simulink model "MdSWReqChk358"  (R2018b)
settings: Solver=FixedStepDiscrete  StartTime=0.0  StopTime=10.0  FixedStep=0.01  RelTol=1e-3
undefined symbols (not defined in the file or in its folder): ChkBsyBitArray4s, ChkBsyBitArray6s7s, KeSMSAutoEZEFwdBkwdPosEna_Val, KeSMSuButtonLongPressedThrshldTm_Val, KeSMSuMdNum4s_Val, KeSMSuMdNum6s7s_Val, SetBsyBitArray4s, SetEnBitArray4s
libraries: RspLib x14, simulink x9
settings Model: Creator=sn2xws  LastModifiedBy=sn55gm
settings Model: ModifiedHistory=|
  | 2023.8.1 CR401790  增加模式21-26的请求
  | V2.1.0
  | 2023.9.18 bug 542961符号方向反了，<= 改为>=
  | V2.3.0
  | 2023.12.28  迎宾向后，条件改为或
  | 2025.2.24 V2.3.1 358MY26车型新增md33，md34，共存模式规则变更
settings DataIOCC: SaveFormat=StructureWithTime
settings OptimizationCC: DefaultParameterBehavior=Inlined  EnhancedBackFolding=on  PassReuseOutputArgsAs=Individual arguments  ZeroExternalMemoryAtStartup=off  ZeroInternalMemoryAtStartup=off  OptimizeBlockOrder=speed  DifferentSizesBufferReuse=on  OptimizationCustomize=off
settings DebuggingCC: ParameterTunabilityLossMsg=error
settings ModelReferenceCC: ModelReferenceNumInstancesAllowed=Single
settings SFSimCC: MATLABDynamicMemAlloc=off
settings RTWCC: SystemTargetFile=autosar.tlc  GenCodeOnly=on  TemplateMakefile=ert_default_tmf  Description=AUTOSAR  GenerateReport=on  IncludeHyperlinkInReport=on  LaunchReport=on  GenerateTraceInfo=on  GenerateTraceReport=on  GenerateTraceReportSl=on  GenerateTraceReportSf=on  GenerateTraceReportEml=on  GenerateCodeMetricsReport=on
settings CodeAppCC: ForceParamTrailComments=on  IgnoreCustomStorageClasses=off  OperatorAnnotations=on  SimulinkDataObjDesc=on  SFDataObjDesc=on  InsertBlockDesc=on
settings STFCustomTargetCC: TargetLangStandard=C99 (ISO)  MultiwordLength=256  ParMdlRefBuildCompliant=on  CompOptLevelCompliant=on  IncludeMdlTerminateFcn=off  CombineOutputUpdateFcns=on  SuppressErrorStatus=on  ERTCustomFileBanners=on  SupportNonFinite=off  SupportComplex=off  SupportContinuousTime=off  SupportNonInlinedSFcns=off  RemoveResetFunc=on  MATLABClassNameForMDSCustomization=Simulink.SoftwareTarget.ERTCustomization  AutosarCompliant=on  UseToolchainInfoCompliant=on  LookupTableObjectStructAxisOrder=2,1,3,4,...  LUTObjectStructOrderEvenSpacing=Size,Table,Breakpoints  SystemTargetFile=autosar.tlc
settings ERTTargetCC: TargetLangStandard=C99 (ISO)  ConcurrentExecutionCompliant=off  IncludeMdlTerminateFcn=off  SuppressErrorStatus=on  SupportNonFinite=off  SupportComplex=off  ModelStepFunctionPrototypeControlCompliant=off  CPPClassGenCompliant=off  AutosarCompliant=on  LookupTableObjectStructAxisOrder=2,1,3,4,...  LUTObjectStructOrderEvenSpacing=Size,Table,Breakpoints  InlinedParameterPlacement=NonHierarchical  ERTCustomFileTemplate=example_file_process.tlc  ERTFilePackagingFormat=Compact

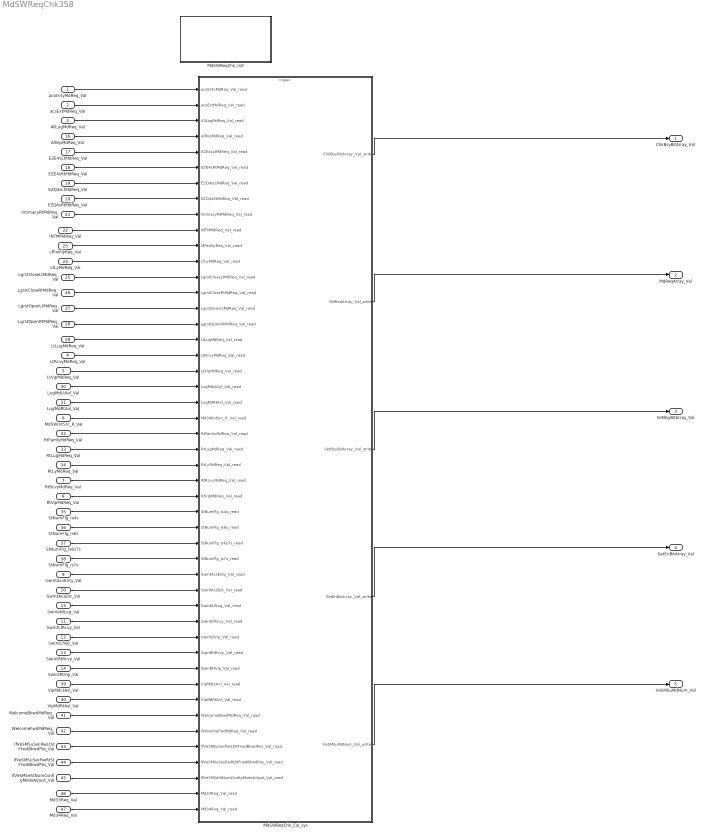
== system MdSWReqChk358 ==
  acsEntyMdReq_Val : Inport  OutDataTypeStr=boolean  PortDimensions=1
  acsExtMdReq_Val : Inport  Port=2  OutDataTypeStr=boolean  PortDimensions=1
  AllLugMdReq_Val : Inport  Port=3  OutDataTypeStr=boolean  PortDimensions=1
  LtRcvyMdReq_Val : Inport  Port=4  OutDataTypeStr=boolean  PortDimensions=1
  LtVipMdReq_Val : Inport  Port=5  OutDataTypeStr=boolean  PortDimensions=1
  MdSWIntSrc_R_Val : Inport  Port=6  OutDataTypeStr=uint16  PortDimensions=1
  RtRcvyMdReq_Val : Inport  Port=7  OutDataTypeStr=boolean  PortDimensions=1
  RtVipMdReq_Val : Inport  Port=8  OutDataTypeStr=boolean  PortDimensions=1
  SwIntAcsEnty_Val : Inport  Port=9  OutDataTypeStr=IntEnable  PortDimensions=1
  SwIntAcsExt_Val : Inport  Port=10  OutDataTypeStr=IntEnable  PortDimensions=1
  SwIntLfRcvy_Val : Inport  Port=11  OutDataTypeStr=IntEnable  PortDimensions=1
  SwIntLfVip_Val : Inport  Port=12  OutDataTypeStr=IntEnable  PortDimensions=1
  SwIntRtRcvy_Val : Inport  Port=13  OutDataTypeStr=IntEnable  PortDimensions=1
  SwIntRtVip_Val : Inport  Port=14  OutDataTypeStr=IntEnable  PortDimensions=1
  SwIntAllLug_Val : Inport  Port=15  OutDataTypeStr=IntEnable  PortDimensions=1
  AllVipMdReq_Val : Inport  Port=16  OutDataTypeStr=boolean  PortDimensions=1
  EZE4sLtMdReq_Val : Inport  Port=17  OutDataTypeStr=boolean  PortDimensions=1
  EZE4sRtMdReq_Val : Inport  Port=18  OutDataTypeStr=boolean  PortDimensions=1
  EZQ4sLtMdReq_Val : Inport  Port=19  OutDataTypeStr=boolean  PortDimensions=1
  EZQ4sRtMdReq_Val : Inport  Port=20  OutDataTypeStr=boolean  PortDimensions=1
  IntimacyRtMdReq_Val : Inport  Port=21  OutDataTypeStr=boolean  PortDimensions=1
  INTMMdReq_Val : Inport  Port=22  OutDataTypeStr=boolean  PortDimensions=1
  LfFamlyReq_Val : Inport  Port=23  OutDataTypeStr=boolean  PortDimensions=1
  LfLyMdReq_Val : Inport  Port=24  OutDataTypeStr=boolean  PortDimensions=1
  LgrstCloseLtMdReq_Val : Inport  Port=25  OutDataTypeStr=boolean  PortDimensions=1
  LgrstCloseRtMdReq_Val : Inport  Port=26  OutDataTypeStr=boolean  PortDimensions=1
  LgrstOpenLtMdReq_Val : Inport  Port=27  OutDataTypeStr=boolean  PortDimensions=1
  LgrstOpenRtMdReq_Val : Inport  Port=28  OutDataTypeStr=boolean  PortDimensions=1
  LtLugMdReq_Val : Inport  Port=29  OutDataTypeStr=boolean  PortDimensions=1
  LugMdLtAvl_Val : Inport  Port=30  OutDataTypeStr=boolean  PortDimensions=1
  LugMdRtAvl_Val : Inport  Port=31  OutDataTypeStr=boolean  PortDimensions=1
  RtFamlyMdReq_Val : Inport  Port=32  OutDataTypeStr=boolean  PortDimensions=1
  RtLugMdReq_Val : Inport  Port=33  OutDataTypeStr=boolean  PortDimensions=1
  RtLyMdReq_Val : Inport  Port=34  OutDataTypeStr=boolean  PortDimensions=1
  StNumFlg_Is4s : Inport  Port=35  OutDataTypeStr=boolean  PortDimensions=1
  StNumFlg_Is6s : Inport  Port=36  OutDataTypeStr=boolean  PortDimensions=1
  StNumFlg_Is6s7s : Inport  Port=37  OutDataTypeStr=boolean  PortDimensions=1
  StNumFlg_Is7s : Inport  Port=38  OutDataTypeStr=boolean  PortDimensions=1
  VipMdLtAvl_Val : Inport  Port=39  OutDataTypeStr=boolean  PortDimensions=1
  VipMdRtAvl_Val : Inport  Port=40  OutDataTypeStr=boolean  PortDimensions=1
  WelcomeBkwdMdReq_Val : Inport  Port=41  OutDataTypeStr=boolean  PortDimensions=1
  WelcomeFwdMdReq_Val : Inport  Port=42  OutDataTypeStr=boolean  PortDimensions=1
  IfVeSMSuSecRwLtStFrwdBkwdPos_Val : Inport  Port=43  OutDataTypeStr=uint16  PortDimensions=1
  IfVeSMSuSecRwRtStFrwdBkwdPos_Val : Inport  Port=44  OutDataTypeStr=uint16  PortDimensions=1
  IfVeSMSeStNumConfigModeAdjust_Val : Inport  Port=45  OutDataTypeStr=uint8  PortDimensions=1
  Md33Req_Val : Inport  Port=46  OutDataTypeStr=boolean  PortDimensions=1
  Md34Req_Val : Inport  Port=47  OutDataTypeStr=boolean  PortDimensions=1
  MdSWReqChk_Cal_sys : Subsystem
  MdSWReqChk_Init : Subsystem
  ChkBsyBitArray_Val : Outport  OutDataTypeStr=uint32  PortDimensions=32
  MdReqArray_Val : Outport  Port=2  OutDataTypeStr=boolean  PortDimensions=32
  SetBsyBitArray_Val : Outport  Port=3  OutDataTypeStr=uint32  PortDimensions=32
  SetEnBitArray_Val : Outport  Port=4  OutDataTypeStr=uint32  PortDimensions=32
  VeSMSuMdNum_Val : Outport  Port=5  OutDataTypeStr=uint8  PortDimensions=1
  wires:
  acsEntyMdReq_Val/1 -> MdSWReqChk_Cal_sys/1(acsEntyMdReq_Val_read)
  acsExtMdReq_Val/1 -> MdSWReqChk_Cal_sys/2(acsExtMdReq_Val_read)
  AllLugMdReq_Val/1 -> MdSWReqChk_Cal_sys/3(AllLugMdReq_Val_read)
  LtRcvyMdReq_Val/1 -> MdSWReqChk_Cal_sys/18(LtRcvyMdReq_Val_read)
  LtVipMdReq_Val/1 -> MdSWReqChk_Cal_sys/19(LtVipMdReq_Val_read)
  MdSWIntSrc_R_Val/1 -> MdSWReqChk_Cal_sys/22(MdSWIntSrc_R_Val_read)
  RtRcvyMdReq_Val/1 -> MdSWReqChk_Cal_sys/26(RtRcvyMdReq_Val_read)
  RtVipMdReq_Val/1 -> MdSWReqChk_Cal_sys/27(RtVipMdReq_Val_read)
  SwIntAcsEnty_Val/1 -> MdSWReqChk_Cal_sys/32(SwIntAcsEnty_Val_read)
  SwIntAcsExt_Val/1 -> MdSWReqChk_Cal_sys/33(SwIntAcsExt_Val_read)
  SwIntLfRcvy_Val/1 -> MdSWReqChk_Cal_sys/35(SwIntLfRcvy_Val_read)
  SwIntLfVip_Val/1 -> MdSWReqChk_Cal_sys/36(SwIntLfVip_Val_read)
  SwIntRtRcvy_Val/1 -> MdSWReqChk_Cal_sys/37(SwIntRtRcvy_Val_read)
  SwIntRtVip_Val/1 -> MdSWReqChk_Cal_sys/38(SwIntRtVip_Val_read)
  SwIntAllLug_Val/1 -> MdSWReqChk_Cal_sys/34(SwIntAllLug_Val_read)
  AllVipMdReq_Val/1 -> MdSWReqChk_Cal_sys/4(AllVipMdReq_Val_read)
  EZE4sLtMdReq_Val/1 -> MdSWReqChk_Cal_sys/5(EZE4sLtMdReq_Val_read)
  EZE4sRtMdReq_Val/1 -> MdSWReqChk_Cal_sys/6(EZE4sRtMdReq_Val_read)
  EZQ4sLtMdReq_Val/1 -> MdSWReqChk_Cal_sys/7(EZQ4sLtMdReq_Val_read)
  EZQ4sRtMdReq_Val/1 -> MdSWReqChk_Cal_sys/8(EZQ4sRtMdReq_Val_read)
  IntimacyRtMdReq_Val/1 -> MdSWReqChk_Cal_sys/9(IntimacyRtMdReq_Val_read)
  INTMMdReq_Val/1 -> MdSWReqChk_Cal_sys/10(INTMMdReq_Val_read)
  LfFamlyReq_Val/1 -> MdSWReqChk_Cal_sys/11(LfFamlyReq_Val_read)
  LfLyMdReq_Val/1 -> MdSWReqChk_Cal_sys/12(LfLyMdReq_Val_read)
  LgrstCloseLtMdReq_Val/1 -> MdSWReqChk_Cal_sys/13(LgrstCloseLtMdReq_Val_read)
  LgrstCloseRtMdReq_Val/1 -> MdSWReqChk_Cal_sys/14(LgrstCloseRtMdReq_Val_read)
  LgrstOpenLtMdReq_Val/1 -> MdSWReqChk_Cal_sys/15(LgrstOpenLtMdReq_Val_read)
  LgrstOpenRtMdReq_Val/1 -> MdSWReqChk_Cal_sys/16(LgrstOpenRtMdReq_Val_read)
  LtLugMdReq_Val/1 -> MdSWReqChk_Cal_sys/17(LtLugMdReq_Val_read)
  LugMdLtAvl_Val/1 -> MdSWReqChk_Cal_sys/20(LugMdLtAvl_Val_read)
  LugMdRtAvl_Val/1 -> MdSWReqChk_Cal_sys/21(LugMdRtAvl_Val_read)
  RtFamlyMdReq_Val/1 -> MdSWReqChk_Cal_sys/23(RtFamlyMdReq_Val_read)
  RtLugMdReq_Val/1 -> MdSWReqChk_Cal_sys/24(RtLugMdReq_Val_read)
  RtLyMdReq_Val/1 -> MdSWReqChk_Cal_sys/25(RtLyMdReq_Val_read)
  StNumFlg_Is4s/1 -> MdSWReqChk_Cal_sys/28(StNumFlg_Is4s_read)
  StNumFlg_Is6s/1 -> MdSWReqChk_Cal_sys/29(StNumFlg_Is6s_read)
  StNumFlg_Is6s7s/1 -> MdSWReqChk_Cal_sys/30(StNumFlg_Is6s7s_read)
  StNumFlg_Is7s/1 -> MdSWReqChk_Cal_sys/31(StNumFlg_Is7s_read)
  VipMdLtAvl_Val/1 -> MdSWReqChk_Cal_sys/39(VipMdLtAvl_Val_read)
  VipMdRtAvl_Val/1 -> MdSWReqChk_Cal_sys/40(VipMdRtAvl_Val_read)
  WelcomeBkwdMdReq_Val/1 -> MdSWReqChk_Cal_sys/41(WelcomeBkwdMdReq_Val_read)
  WelcomeFwdMdReq_Val/1 -> MdSWReqChk_Cal_sys/42(WelcomeFwdMdReq_Val_read)
  MdSWReqChk_Cal_sys/1(ChkBsyBitArray_Val_write) -> ChkBsyBitArray_Val/1
  MdSWReqChk_Cal_sys/2(MdReqArray_Val_write) -> MdReqArray_Val/1
  MdSWReqChk_Cal_sys/3(SetBsyBitArray_Val_write) -> SetBsyBitArray_Val/1
  MdSWReqChk_Cal_sys/4(SetEnBitArray_Val_write) -> SetEnBitArray_Val/1
  MdSWReqChk_Cal_sys/5(VeSMSuMdNum_Val_write) -> VeSMSuMdNum_Val/1
  IfVeSMSuSecRwLtStFrwdBkwdPos_Val/1 -> MdSWReqChk_Cal_sys/43(IfVeSMSuSecRwLtStFrwdBkwdPos_Val_read)
  IfVeSMSuSecRwRtStFrwdBkwdPos_Val/1 -> MdSWReqChk_Cal_sys/44(IfVeSMSuSecRwRtStFrwdBkwdPos_Val_read)
  IfVeSMSeStNumConfigModeAdjust_Val/1 -> MdSWReqChk_Cal_sys/45(IfVeSMSeStNumConfigModeAdjust_Val_read)
  Md33Req_Val/1 -> MdSWReqChk_Cal_sys/46(Md33Req_Val_read)
  Md34Req_Val/1 -> MdSWReqChk_Cal_sys/47(Md34Req_Val_read)

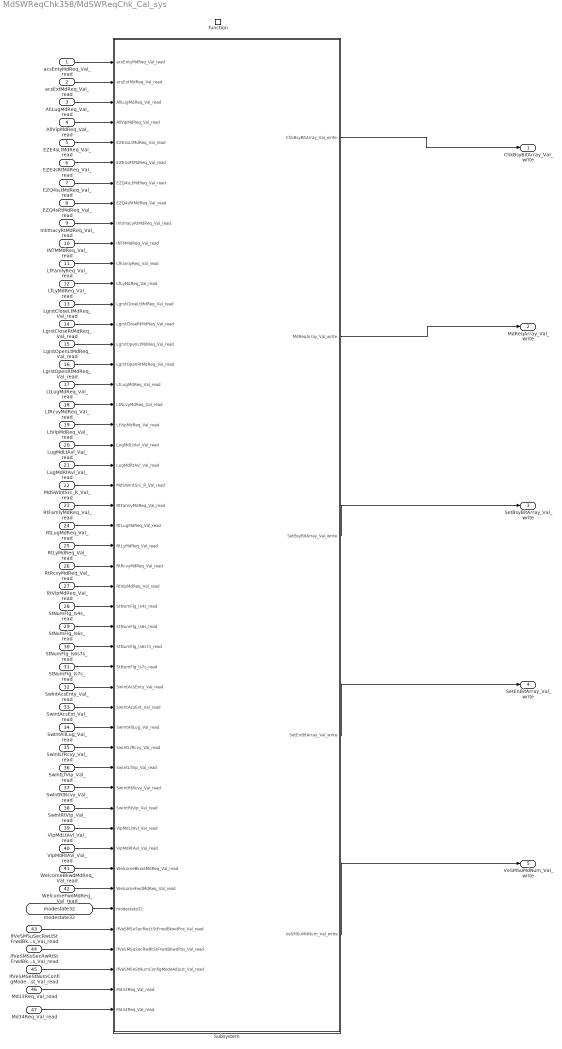
== system MdSWReqChk358/MdSWReqChk_Cal_sys ==
  acsEntyMdReq_Val_read : Inport
  acsExtMdReq_Val_read : Inport  Port=2
  AllLugMdReq_Val_read : Inport  Port=3
  AllVipMdReq_Val_read : Inport  Port=4
  EZE4sLtMdReq_Val_read : Inport  Port=5
  EZE4sRtMdReq_Val_read : Inport  Port=6
  EZQ4sLtMdReq_Val_read : Inport  Port=7
  EZQ4sRtMdReq_Val_read : Inport  Port=8
  IntimacyRtMdReq_Val_read : Inport  Port=9
  INTMMdReq_Val_read : Inport  Port=10
  LfFamlyReq_Val_read : Inport  Port=11
  LfLyMdReq_Val_read : Inport  Port=12
  LgrstCloseLtMdReq_Val_read : Inport  Port=13
  LgrstCloseRtMdReq_Val_read : Inport  Port=14
  LgrstOpenLtMdReq_Val_read : Inport  Port=15
  LgrstOpenRtMdReq_Val_read : Inport  Port=16
  LtLugMdReq_Val_read : Inport  Port=17
  LtRcvyMdReq_Val_read : Inport  Port=18
  LtVipMdReq_Val_read : Inport  Port=19
  LugMdLtAvl_Val_read : Inport  Port=20
  LugMdRtAvl_Val_read : Inport  Port=21
  MdSWIntSrc_R_Val_read : Inport  Port=22
  RtFamlyMdReq_Val_read : Inport  Port=23
  RtLugMdReq_Val_read : Inport  Port=24
  RtLyMdReq_Val_read : Inport  Port=25
  RtRcvyMdReq_Val_read : Inport  Port=26
  RtVipMdReq_Val_read : Inport  Port=27
  StNumFlg_Is4s_read : Inport  Port=28
  StNumFlg_Is6s_read : Inport  Port=29
  StNumFlg_Is6s7s_read : Inport  Port=30
  StNumFlg_Is7s_read : Inport  Port=31
  SwIntAcsEnty_Val_read : Inport  Port=32
  SwIntAcsExt_Val_read : Inport  Port=33
  SwIntAllLug_Val_read : Inport  Port=34
  SwIntLfRcvy_Val_read : Inport  Port=35
  SwIntLfVip_Val_read : Inport  Port=36
  SwIntRtRcvy_Val_read : Inport  Port=37
  SwIntRtVip_Val_read : Inport  Port=38
  VipMdLtAvl_Val_read : Inport  Port=39
  VipMdRtAvl_Val_read : Inport  Port=40
  WelcomeBkwdMdReq_Val_read : Inport  Port=41
  WelcomeFwdMdReq_Val_read : Inport  Port=42
  IfVeSMSuSecRwLtStFrwdBkwdPos_Val_read : Inport  Port=43
  IfVeSMSuSecRwRtStFrwdBkwdPos_Val_read : Inport  Port=44
  IfVeSMSeStNumConfigModeAdjust_Val_read : Inport  Port=45
  Md33Req_Val_read : Inport  Port=46
  Md34Req_Val_read : Inport  Port=47
  function : TriggerPort  TriggerType=function-call  IsSimulinkFunction=on  FunctionName=MdSWReqChk_Cal  VariantControl=(inherit)
  Subsystem : Subsystem
  modestate32 : ArgIn  OutDataTypeStr=uint32  ArgumentName=modestate32
  ChkBsyBitArray_Val_write : Outport
      settings: EnsureOutportIsVirtual=on
  MdReqArray_Val_write : Outport  Port=2
      settings: EnsureOutportIsVirtual=on
  SetBsyBitArray_Val_write : Outport  Port=3
      settings: EnsureOutportIsVirtual=on
  SetEnBitArray_Val_write : Outport  Port=4
      settings: EnsureOutportIsVirtual=on
  VeSMSuMdNum_Val_write : Outport  Port=5
      settings: EnsureOutportIsVirtual=on
  wires:
  acsEntyMdReq_Val_read/1 -> Subsystem/1(acsEntyMdReq_Val_read)
  acsExtMdReq_Val_read/1 -> Subsystem/2(acsExtMdReq_Val_read)
  AllLugMdReq_Val_read/1 -> Subsystem/3(AllLugMdReq_Val_read)
  AllVipMdReq_Val_read/1 -> Subsystem/4(AllVipMdReq_Val_read)
  EZE4sLtMdReq_Val_read/1 -> Subsystem/5(EZE4sLtMdReq_Val_read)
  EZE4sRtMdReq_Val_read/1 -> Subsystem/6(EZE4sRtMdReq_Val_read)
  EZQ4sLtMdReq_Val_read/1 -> Subsystem/7(EZQ4sLtMdReq_Val_read)
  EZQ4sRtMdReq_Val_read/1 -> Subsystem/8(EZQ4sRtMdReq_Val_read)
  IntimacyRtMdReq_Val_read/1 -> Subsystem/9(IntimacyRtMdReq_Val_read)
  INTMMdReq_Val_read/1 -> Subsystem/10(INTMMdReq_Val_read)
  LfFamlyReq_Val_read/1 -> Subsystem/11(LfFamlyReq_Val_read)
  LfLyMdReq_Val_read/1 -> Subsystem/12(LfLyMdReq_Val_read)
  LgrstCloseLtMdReq_Val_read/1 -> Subsystem/13(LgrstCloseLtMdReq_Val_read)
  LgrstCloseRtMdReq_Val_read/1 -> Subsystem/14(LgrstCloseRtMdReq_Val_read)
  LgrstOpenLtMdReq_Val_read/1 -> Subsystem/15(LgrstOpenLtMdReq_Val_read)
  LgrstOpenRtMdReq_Val_read/1 -> Subsystem/16(LgrstOpenRtMdReq_Val_read)
  LtLugMdReq_Val_read/1 -> Subsystem/17(LtLugMdReq_Val_read)
  LtRcvyMdReq_Val_read/1 -> Subsystem/18(LtRcvyMdReq_Val_read)
  LtVipMdReq_Val_read/1 -> Subsystem/19(LtVipMdReq_Val_read)
  LugMdLtAvl_Val_read/1 -> Subsystem/20(LugMdLtAvl_Val_read)
  LugMdRtAvl_Val_read/1 -> Subsystem/21(LugMdRtAvl_Val_read)
  MdSWIntSrc_R_Val_read/1 -> Subsystem/22(MdSWIntSrc_R_Val_read)
  RtFamlyMdReq_Val_read/1 -> Subsystem/23(RtFamlyMdReq_Val_read)
  RtLugMdReq_Val_read/1 -> Subsystem/24(RtLugMdReq_Val_read)
  RtLyMdReq_Val_read/1 -> Subsystem/25(RtLyMdReq_Val_read)
  RtRcvyMdReq_Val_read/1 -> Subsystem/26(RtRcvyMdReq_Val_read)
  RtVipMdReq_Val_read/1 -> Subsystem/27(RtVipMdReq_Val_read)
  StNumFlg_Is4s_read/1 -> Subsystem/28(StNumFlg_Is4s_read)
  StNumFlg_Is6s_read/1 -> Subsystem/29(StNumFlg_Is6s_read)
  StNumFlg_Is6s7s_read/1 -> Subsystem/30(StNumFlg_Is6s7s_read)
  StNumFlg_Is7s_read/1 -> Subsystem/31(StNumFlg_Is7s_read)
  SwIntAcsEnty_Val_read/1 -> Subsystem/32(SwIntAcsEnty_Val_read)
  SwIntAcsExt_Val_read/1 -> Subsystem/33(SwIntAcsExt_Val_read)
  SwIntAllLug_Val_read/1 -> Subsystem/34(SwIntAllLug_Val_read)
  SwIntLfRcvy_Val_read/1 -> Subsystem/35(SwIntLfRcvy_Val_read)
  SwIntLfVip_Val_read/1 -> Subsystem/36(SwIntLfVip_Val_read)
  SwIntRtRcvy_Val_read/1 -> Subsystem/37(SwIntRtRcvy_Val_read)
  SwIntRtVip_Val_read/1 -> Subsystem/38(SwIntRtVip_Val_read)
  VipMdLtAvl_Val_read/1 -> Subsystem/39(VipMdLtAvl_Val_read)
  VipMdRtAvl_Val_read/1 -> Subsystem/40(VipMdRtAvl_Val_read)
  WelcomeBkwdMdReq_Val_read/1 -> Subsystem/41(WelcomeBkwdMdReq_Val_read)
  WelcomeFwdMdReq_Val_read/1 -> Subsystem/42(WelcomeFwdMdReq_Val_read)
  Subsystem/1(ChkBsyBitArray_Val_write) -> ChkBsyBitArray_Val_write/1
  Subsystem/2(MdReqArray_Val_write) -> MdReqArray_Val_write/1
  Subsystem/3(SetBsyBitArray_Val_write) -> SetBsyBitArray_Val_write/1
  Subsystem/4(SetEnBitArray_Val_write) -> SetEnBitArray_Val_write/1
  modestate32/1 -> Subsystem/43(modestate32)
  Subsystem/5(VeSMSuMdNum_Val_write) -> VeSMSuMdNum_Val_write/1
  IfVeSMSuSecRwLtStFrwdBkwdPos_Val_read/1 -> Subsystem/44(IfVeSMSuSecRwLtStFrwdBkwdPos_Val_read)
  IfVeSMSuSecRwRtStFrwdBkwdPos_Val_read/1 -> Subsystem/45(IfVeSMSuSecRwRtStFrwdBkwdPos_Val_read)
  IfVeSMSeStNumConfigModeAdjust_Val_read/1 -> Subsystem/46(IfVeSMSeStNumConfigModeAdjust_Val_read)
  Md33Req_Val_read/1 -> Subsystem/47(Md33Req_Val_read)
  Md34Req_Val_read/1 -> Subsystem/48(Md34Req_Val_read)

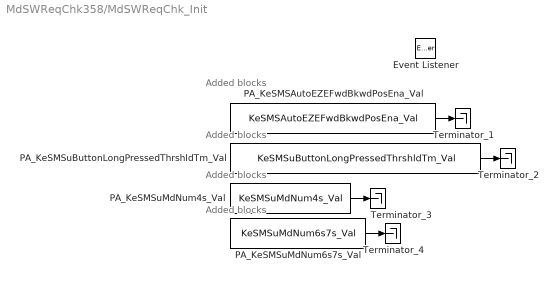
== system MdSWReqChk358/MdSWReqChk_Init ==
  note: Added blocks
  note: Added blocks
  note: Added blocks
  note: Added blocks
  Event Listener : EventListener  EventName=reset
  PA_KeSMSAutoEZEFwdBkwdPosEna_Val : Constant  Value=KeSMSAutoEZEFwdBkwdPosEna_Val
  PA_KeSMSuButtonLongPressedThrshldTm_Val : Constant  Value=KeSMSuButtonLongPressedThrshldTm_Val
  PA_KeSMSuMdNum4s_Val : Constant  Value=KeSMSuMdNum4s_Val
  PA_KeSMSuMdNum6s7s_Val : Constant  Value=KeSMSuMdNum6s7s_Val
  Terminator_{1..4} (4 alike) : Terminator
  wires:
  PA_KeSMSAutoEZEFwdBkwdPosEna_Val/1 -> Terminator_1/1
  PA_KeSMSuButtonLongPressedThrshldTm_Val/1 -> Terminator_2/1
  PA_KeSMSuMdNum4s_Val/1 -> Terminator_3/1
  PA_KeSMSuMdNum6s7s_Val/1 -> Terminator_4/1

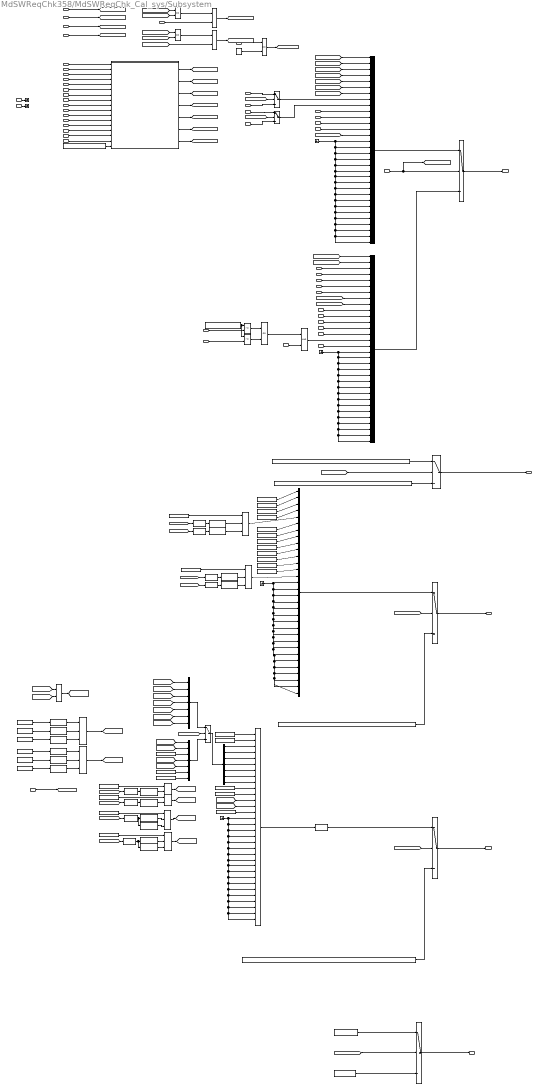
== system MdSWReqChk358/MdSWReqChk_Cal_sys/Subsystem ==
  note: 2023.12.28 迎宾向后，条件改为或
  note: bug542961
  note: 符号方向反了，<= 改为>=
  note: 2023.8.1 CR401790 增加模式21-26的请求
  note: VIPR
  note: RcvyR
  note: VIPL
  note: LugL
  note: LugR
  note: RcvyL
  acsEntyMdReq_Val_read : Inport
  acsExtMdReq_Val_read : Inport  Port=2
  AllLugMdReq_Val_read : Inport  Port=3
  AllVipMdReq_Val_read : Inport  Port=4
  EZE4sLtMdReq_Val_read : Inport  Port=5
  EZE4sRtMdReq_Val_read : Inport  Port=6
  EZQ4sLtMdReq_Val_read : Inport  Port=7
  EZQ4sRtMdReq_Val_read : Inport  Port=8
  IntimacyRtMdReq_Val_read : Inport  Port=9
  INTMMdReq_Val_read : Inport  Port=10
  LfFamlyReq_Val_read : Inport  Port=11
  LfLyMdReq_Val_read : Inport  Port=12
  LgrstCloseLtMdReq_Val_read : Inport  Port=13
  LgrstCloseRtMdReq_Val_read : Inport  Port=14
  LgrstOpenLtMdReq_Val_read : Inport  Port=15
  LgrstOpenRtMdReq_Val_read : Inport  Port=16
  LtLugMdReq_Val_read : Inport  Port=17
  LtRcvyMdReq_Val_read : Inport  Port=18
  LtVipMdReq_Val_read : Inport  Port=19
  LugMdLtAvl_Val_read : Inport  Port=20
  LugMdRtAvl_Val_read : Inport  Port=21
  MdSWIntSrc_R_Val_read : Inport  Port=22
  RtFamlyMdReq_Val_read : Inport  Port=23
  RtLugMdReq_Val_read : Inport  Port=24
  RtLyMdReq_Val_read : Inport  Port=25
  RtRcvyMdReq_Val_read : Inport  Port=26
  RtVipMdReq_Val_read : Inport  Port=27
  StNumFlg_Is4s_read : Inport  Port=28
  StNumFlg_Is6s_read : Inport  Port=29
  StNumFlg_Is6s7s_read : Inport  Port=30
  StNumFlg_Is7s_read : Inport  Port=31
  SwIntAcsEnty_Val_read : Inport  Port=32
  SwIntAcsExt_Val_read : Inport  Port=33
  SwIntAllLug_Val_read : Inport  Port=34
  SwIntLfRcvy_Val_read : Inport  Port=35
  SwIntLfVip_Val_read : Inport  Port=36
  SwIntRtRcvy_Val_read : Inport  Port=37
  SwIntRtVip_Val_read : Inport  Port=38
  VipMdLtAvl_Val_read : Inport  Port=39
  VipMdRtAvl_Val_read : Inport  Port=40
  WelcomeBkwdMdReq_Val_read : Inport  Port=41
  WelcomeFwdMdReq_Val_read : Inport  Port=42
  modestate32 : Inport  Port=43
  IfVeSMSuSecRwLtStFrwdBkwdPos_Val_read : Inport  Port=44
  IfVeSMSuSecRwRtStFrwdBkwdPos_Val_read : Inport  Port=45
  IfVeSMSeStNumConfigModeAdjust_Val_read : Inport  Port=46
  Md33Req_Val_read : Inport  Port=47
  Md34Req_Val_read : Inport  Port=48
  Bitwise Operator{,1,4..7} (6 alike) : simulink/Logic and Bit Operations/Bitwise Operator  logicop=OR  UseBitMask=off  NumInputPorts=3  BitMask=bin2dec('11011001')  BitMaskRealWorld=Stored Integer
  Bitwise Operator2 : simulink/Logic and Bit Operations/Bitwise Operator  logicop=OR  UseBitMask=off  NumInputPorts=2  BitMask=bin2dec('11011001')  BitMaskRealWorld=Stored Integer
  Bitwise Operator3 : simulink/Logic and Bit Operations/Bitwise Operator  logicop=OR  UseBitMask=off  NumInputPorts=2  BitMask=bin2dec('11011001')  BitMaskRealWorld=Stored Integer
  Bitwise Operator8 : simulink/Logic and Bit Operations/Bitwise Operator  logicop=OR  UseBitMask=off  NumInputPorts=2  BitMask=bin2dec('11011001')  BitMaskRealWorld=Stored Integer
  Constant : Constant  Value=ChkBsyBitArray6s7s  OutDataTypeStr=uint32
  Constant1 : Constant  Value=ChkBsyBitArray4s  OutDataTypeStr=uint32
  Constant{4..6,8..10,39} (7 alike) : Constant  OutDataTypeStr=uint32
  Constant2 : Constant  Value=SetEnBitArray4s  OutDataTypeStr=uint32
  Constant26 : Constant  Value=8  OutDataTypeStr=uint32
  Constant27 : Constant  Value=512  OutDataTypeStr=uint32
  Constant28 : Constant  Value=2048  OutDataTypeStr=uint32
  Constant29 : Constant  Value=2  OutDataTypeStr=uint32
  Constant3 : Constant  Value=4
  Constant30 : Constant  Value=1024  OutDataTypeStr=uint32
  Constant31 : Constant  Value=4096  OutDataTypeStr=uint32
  Constant32 : Constant  Value=64  OutDataTypeStr=uint32
  Constant33 : Constant  Value=32  OutDataTypeStr=uint32
  Constant34 : Constant  Value=16  OutDataTypeStr=uint32
  Constant35 : Constant  Value=524288  OutDataTypeStr=uint32
  Constant36 : Constant  Value=128  OutDataTypeStr=uint32
  Constant37 : Constant  Value=256  OutDataTypeStr=uint32
  Constant38 : Constant  Value=4  OutDataTypeStr=uint32
  Constant{40..41,44..49} (8 alike) : Constant  Value=532479  OutDataTypeStr=uint32
  Constant42 : Constant  Value=526079  OutDataTypeStr=uint32
  Constant43 : Constant  Value=530815  OutDataTypeStr=uint32
  Constant50 : Constant  Value=526079  OutDataTypeStr=uint32
  Constant51 : Constant  Value=530815  OutDataTypeStr=uint32
  Constant7 : Constant  Value=SetBsyBitArray4s  OutDataTypeStr=uint32
  Data Type Conversion{,1..7} (8 alike) : DataTypeConversion  OutDataTypeStr=uint32
  Data Type Conversion11 : DataTypeConversion
  Demux : Demux  Outputs=7
  Ground{,1..3} (4 alike) : Ground
  Logical Operator : Logic  Operator=OR  AllPortsSameDT=off  OutDataTypeStr=boolean
  Logical Operator1 : Logic  AllPortsSameDT=off  OutDataTypeStr=boolean
  Logical Operator2 : Logic  Operator=OR  AllPortsSameDT=off  OutDataTypeStr=boolean
  Logical Operator3 : Logic  AllPortsSameDT=off  OutDataTypeStr=boolean
  Logical Operator4 : Logic  Operator=OR  AllPortsSameDT=off  OutDataTypeStr=boolean
  Logical Operator5 : Logic  AllPortsSameDT=off  OutDataTypeStr=boolean
  Mux{,1..3} (4 alike) : Mux  Inputs=32
  Mux4 : Mux  Inputs=7
  Mux5 : Mux  Inputs=7
  PA_KeSMSAutoEZEFwdBkwdPosEna_Val : Constant  Value=KeSMSAutoEZEFwdBkwdPosEna_Val
  PA_KeSMSuButtonLongPressedThrshldTm_Val : Constant  Value=KeSMSuButtonLongPressedThrshldTm_Val
  PA_KeSMSuMdNum4s_Val : Constant  Value=KeSMSuMdNum4s_Val
  PA_KeSMSuMdNum6s7s_Val : Constant  Value=KeSMSuMdNum6s7s_Val
  Relational Operator : RelationalOperator  OutDataTypeStr=boolean  RndMeth=Simplest
  Relational Operator1 : RelationalOperator  OutDataTypeStr=boolean  RndMeth=Simplest
  Relational Operator2 : RelationalOperator  Operator===  OutDataTypeStr=boolean  RndMeth=Simplest
  Shift Arithmetic : ArithShift  BitShiftNumber=9  BitShiftDirection=Left
  Shift Arithmetic1 : ArithShift  BitShiftNumber=11  BitShiftDirection=Left
  Shift Arithmetic10 : ArithShift  BitShiftNumber=10  BitShiftDirection=Left
  Shift Arithmetic11 : ArithShift  BitShiftNumber=9  BitShiftDirection=Left
  Shift Arithmetic12 : ArithShift  BitShiftNumber=5  BitShiftDirection=Left
  Shift Arithmetic13 : ArithShift  BitShiftNumber=6  BitShiftDirection=Left
  Shift Arithmetic14 : ArithShift  BitShiftNumber=11  BitShiftDirection=Left
  Shift Arithmetic15 : ArithShift  BitShiftNumber=12  BitShiftDirection=Left
  Shift Arithmetic2 : ArithShift  BitShiftNumber=7  BitShiftDirection=Left
  Shift Arithmetic3 : ArithShift  BitShiftNumber=8  BitShiftDirection=Left
  Shift Arithmetic4 : ArithShift  BitShiftNumber=8  BitShiftDirection=Left
  Shift Arithmetic5 : ArithShift  BitShiftNumber=7  BitShiftDirection=Left
  Shift Arithmetic6 : ArithShift  BitShiftNumber=12  BitShiftDirection=Left
  Shift Arithmetic7 : ArithShift  BitShiftNumber=10  BitShiftDirection=Left
  Shift Arithmetic8 : ArithShift  BitShiftNumber=11  BitShiftDirection=Left
  Shift Arithmetic9 : ArithShift  BitShiftNumber=9  BitShiftDirection=Left
  Subsystem : Subsystem
  Switch{,1..7} (8 alike) : Switch  Criteria=u2 > Threshold
  Terminator_28 : Terminator
  Terminator_29 : Terminator
  ChkBsyBitArray_Val_write : Outport
      settings: EnsureOutportIsVirtual=on
  MdReqArray_Val_write : Outport  Port=2
      settings: EnsureOutportIsVirtual=on
  SetBsyBitArray_Val_write : Outport  Port=3
      settings: EnsureOutportIsVirtual=on
  SetEnBitArray_Val_write : Outport  Port=4
      settings: EnsureOutportIsVirtual=on
  VeSMSuMdNum_Val_write : Outport  Port=5
      settings: EnsureOutportIsVirtual=on
  wires:
  StNumFlg_Is4s_read/1 -> Terminator_28/1
  StNumFlg_Is7s_read/1 -> [is7s]
  PA_KeSMSuButtonLongPressedThrshldTm_Val/1 -> Subsystem/17(KeSMSuButtonLongPressedThrshldTm_Val)
  StNumFlg_Is6s_read/1 -> Terminator_29/1
  modestate32/1 -> Subsystem/7(modestate32_Val_read)
  acsEntyMdReq_Val_read/1 -> Subsystem/1(acsEntyMdReq_Val_read)
  AllLugMdReq_Val_read/1 -> Subsystem/3(AllLugMdReq_Val_read)
  acsExtMdReq_Val_read/1 -> Subsystem/2(acsExtMdReq_Val_read)
  MdSWIntSrc_R_Val_read/1 -> Subsystem/6(MdSWIntSrc_R_Val_read)
  LtVipMdReq_Val_read/1 -> Subsystem/5(LtVipMdReq_Val_read)
  LtRcvyMdReq_Val_read/1 -> Subsystem/4(LtRcvyMdReq_Val_read)
  RtRcvyMdReq_Val_read/1 -> Subsystem/8(RtRcvyMdReq_Val_read)
  RtVipMdReq_Val_read/1 -> Subsystem/9(RtVipMdReq_Val_read)
  SwIntAcsEnty_Val_read/1 -> Subsystem/10(SwIntAcsEnty_Val_read)
  SwIntAcsExt_Val_read/1 -> Subsystem/11(SwIntAcsExt_Val_read)
  SwIntLfRcvy_Val_read/1 -> Subsystem/12(SwIntLfRcvy_Val_read)
  SwIntLfVip_Val_read/1 -> Subsystem/13(SwIntLfVip_Val_read)
  SwIntRtVip_Val_read/1 -> Subsystem/15(SwIntRtVip_Val_read)
  SwIntAllLug_Val_read/1 -> Subsystem/16(SwIntAllLug_Val_read)
  SwIntRtRcvy_Val_read/1 -> Subsystem/14(SwIntRtRcvy_Val_read)
  Subsystem/1(acsEntyMdReqChk_Val_write) -> [EZEReq]
  Subsystem/2(acsExtMdReqChk_Val_write) -> [EZQReq]
  Subsystem/3(AllLugMdReqChk_Val_write) -> [AllLugReq]
  Subsystem/4(LtRcvyMdReqChk_Val_write) -> [LtRcvyReq]
  Subsystem/5(LtVipMdReqChk_Val_write) -> [LtVIPReq]
  Subsystem/6(RtRcvyMdReqChk_Val_write) -> [RtRcvyReq]
  Subsystem/7(RtVipMdReqChk_Val_write) -> [RtVIPReq]
  [EZEReq] -> Mux/1
  [EZQReq] -> Mux/2
  [LtVIPReq] -> Mux/3
  [RtVIPReq] -> Mux/4
  VipMdLtAvl_Val_read/1 -> [VipLtAvl]
  VipMdRtAvl_Val_read/1 -> [VipRtAvl]
  [VipLtAvl] -> Logical Operator/1
  [VipRtAvl] -> Logical Operator/2
  Logical Operator/1 -> Logical Operator1/1
  AllVipMdReq_Val_read/1 -> Logical Operator1/2
  Logical Operator1/1 -> [AllVipReq]
  [AllVipReq] -> Mux/5
  [LtRcvyReq] -> Mux/6
  [RtRcvyReq] -> Mux/7
  INTMMdReq_Val_read/1 -> Mux/10
  IntimacyRtMdReq_Val_read/1 -> Mux/11
  LtLugMdReq_Val_read/1 -> Mux/12
  RtLugMdReq_Val_read/1 -> Mux/13
  Logical Operator3/1 -> [AllLugReqComfirm]
  [AllLugReq] -> Logical Operator3/2
  Logical Operator2/1 -> Logical Operator3/1
  LugMdLtAvl_Val_read/1 -> [LugLtAvl]
  LugMdRtAvl_Val_read/1 -> [LugRtAvl]
  [LugLtAvl] -> Logical Operator2/1
  [LugRtAvl] -> Logical Operator2/2
  [AllLugReqComfirm] -> Mux/14
  Switch/1 -> MdReqArray_Val_write/1
  StNumFlg_Is6s7s_read/1 -> [Is6s7s], Switch/2
  Mux/1 -> Switch/1
  Ground/1 -> Mux/32, Mux/31, Mux/30, Mux/29, Mux/28, Mux/27, Mux/26, Mux/25, Mux/24, Mux/23, Mux/22, Mux/21, Mux/20, Mux/19, Mux/18, Mux/17, Mux/16, Mux/15
  [LtVIPReq] -> Mux1/1
  [LtRcvyReq] -> Mux1/2
  LfLyMdReq_Val_read/1 -> Mux1/3
  LgrstOpenLtMdReq_Val_read/1 -> Mux1/4
  LgrstCloseLtMdReq_Val_read/1 -> Mux1/5
  EZE4sLtMdReq_Val_read/1 -> Mux1/6
  EZQ4sLtMdReq_Val_read/1 -> Mux1/7
  [RtVIPReq] -> Mux1/8
  [RtRcvyReq] -> Mux1/9
  RtLyMdReq_Val_read/1 -> Mux1/10
  LgrstOpenRtMdReq_Val_read/1 -> Mux1/11
  LgrstCloseRtMdReq_Val_read/1 -> Mux1/12
  EZE4sRtMdReq_Val_read/1 -> Mux1/13
  EZQ4sRtMdReq_Val_read/1 -> Mux1/14
  WelcomeFwdMdReq_Val_read/1 -> Mux1/16
  Ground1/1 -> Mux1/27, Mux1/28, Mux1/32, Mux1/31, Mux1/30, Mux1/29, Mux1/26, Mux1/25, Mux1/24, Mux1/23, Mux1/22, Mux1/21, Mux1/20, Mux1/19, Mux1/18, Mux1/17
  Mux1/1 -> Switch/3
  [Is6s7s] -> Switch1/2
  Switch1/1 -> ChkBsyBitArray_Val_write/1
  Constant/1 -> Switch1/1
  Constant1/1 -> Switch1/3
  Constant2/1 -> Switch2/3
  [Is6s7s] -> Switch2/2
  Constant33/1 -> Mux2/9
  Mux2/1 -> Switch2/1  "SetEnBitArray"
  Data Type Conversion/1 -> Shift Arithmetic/1
  Constant37/1 -> Mux2/13
  Constant39/1 -> Mux2/1
  [VipRtAvl] -> Data Type Conversion1/1
  Constant28/1 -> Mux2/4
  Constant26/1 -> Mux2/2
  Bitwise Operator/1 -> Mux2/5
  Constant32/1 -> Mux2/8
  Constant30/1 -> Mux2/6
  Bitwise Operator1/1 -> Mux2/14
  Constant35/1 -> Mux2/11
  [VipLtAvl] -> Data Type Conversion/1
  Constant31/1 -> Mux2/7
  Constant34/1 -> Mux2/10
  Constant36/1 -> Mux2/12
  Constant29/1 -> Bitwise Operator/1
  [LugLtAvl] -> Data Type Conversion2/1
  Shift Arithmetic/1 -> Bitwise Operator/2
  Constant27/1 -> Mux2/3
  Data Type Conversion1/1 -> Shift Arithmetic1/1
  Constant38/1 -> Bitwise Operator1/1
  Shift Arithmetic1/1 -> Bitwise Operator/3
  Data Type Conversion2/1 -> Shift Arithmetic2/1
  Shift Arithmetic2/1 -> Bitwise Operator1/2
  [LugRtAvl] -> Data Type Conversion3/1
  Data Type Conversion3/1 -> Shift Arithmetic3/1
  Shift Arithmetic3/1 -> Bitwise Operator1/3
  Switch2/1 -> SetEnBitArray_Val_write/1
  Ground2/1 -> Mux2/18, Mux2/19, Mux2/20, Mux2/22, Mux2/23, Mux2/32, Mux2/31, Mux2/30, Mux2/29, Mux2/28, Mux2/27, Mux2/26, Mux2/25, Mux2/24, Mux2/21, Mux2/17, Mux2/16, Mux2/15
  Switch3/1 -> SetBsyBitArray_Val_write/1
  [Is6s7s] -> Switch3/2
  Constant7/1 -> Switch3/3
  Constant47/1 -> Mux3/10
  Data Type Conversion11/1 -> Switch3/1  "SetBsyBitArray"
  Constant49/1 -> Mux3/14
  Constant40/1 -> Mux3/1
  [RghtBsyBit2] -> Mux3/13
  Constant48/1 -> Mux3/11
  Constant41/1 -> Mux3/2
  [LftBsyBit2] -> Mux3/12
  Mux3/1 -> Data Type Conversion11/1
  [is7s] -> Data Type Conversion5/1
  Shift Arithmetic8/1 -> Bitwise Operator4/3
  Constant50/1 -> Bitwise Operator4/1
  [is7s] -> Data Type Conversion7/1
  Shift Arithmetic4/1 -> Bitwise Operator2/2
  [is7s] -> Data Type Conversion6/1
  Data Type Conversion4/1 -> Shift Arithmetic4/1
  [is7s] -> Data Type Conversion4/1
  Shift Arithmetic9/1 -> Bitwise Operator5/3
  Constant51/1 -> Bitwise Operator5/1
  Bitwise Operator3/1 -> [RghtBsyBit]
  Data Type Conversion7/1 -> Shift Arithmetic9/1, Shift Arithmetic7/1
  Bitwise Operator4/1 -> [LftBsyBit2]
  Shift Arithmetic6/1 -> Bitwise Operator4/2
  Data Type Conversion5/1 -> Shift Arithmetic5/1
  Constant42/1 -> Bitwise Operator2/1
  Data Type Conversion6/1 -> Shift Arithmetic8/1, Shift Arithmetic6/1
  Bitwise Operator5/1 -> [RghtBsyBit2]
  Shift Arithmetic5/1 -> Bitwise Operator3/2
  Bitwise Operator2/1 -> [LftBsyBit]
  Constant43/1 -> Bitwise Operator3/1
  Shift Arithmetic7/1 -> Bitwise Operator5/2
  Ground3/1 -> Mux3/32, Mux3/31, Mux3/30, Mux3/29, Mux3/28, Mux3/27, Mux3/26, Mux3/25, Mux3/24, Mux3/23, Mux3/22, Mux3/21, Mux3/20, Mux3/19, Mux3/18, Mux3/17, Mux3/16, Mux3/15
  [Is6s7s] -> Switch4/2
  PA_KeSMSuMdNum4s_Val/1 -> Switch4/3
  PA_KeSMSuMdNum6s7s_Val/1 -> Switch4/1  "SetBsyBitArray"
  Switch4/1 -> VeSMSuMdNum_Val_write/1
  PA_KeSMSAutoEZEFwdBkwdPosEna_Val/1 -> Relational Operator1/1, Relational Operator/1
  IfVeSMSuSecRwLtStFrwdBkwdPos_Val_read/1 -> Relational Operator/2
  IfVeSMSuSecRwRtStFrwdBkwdPos_Val_read/1 -> Relational Operator1/2
  Relational Operator/1 -> Logical Operator4/1
  Relational Operator1/1 -> Logical Operator4/2
  Logical Operator5/1 -> Mux1/15
  WelcomeBkwdMdReq_Val_read/1 -> Logical Operator5/2
  Logical Operator4/1 -> Logical Operator5/1
  IfVeSMSeStNumConfigModeAdjust_Val_read/1 -> Relational Operator2/1
  Constant3/1 -> Relational Operator2/2
  Relational Operator2/1 -> [Is3582]
  [Is3582] -> Switch5/2
  Md34Req_Val_read/1 -> Switch5/1
  LfFamlyReq_Val_read/1 -> Switch5/3
  Switch5/1 -> Mux/8
  Switch6/1 -> Mux/9
  [Is3582] -> Switch6/2
  Md33Req_Val_read/1 -> Switch6/1
  RtFamlyMdReq_Val_read/1 -> Switch6/3
  Constant4/1 -> Shift Arithmetic10/1
  Constant5/1 -> Shift Arithmetic11/1
  Shift Arithmetic10/1 -> Bitwise Operator6/1
  Shift Arithmetic11/1 -> Bitwise Operator6/2
  Bitwise Operator6/1 -> [LftBsyBit3582]
  Shift Arithmetic12/1 -> Bitwise Operator6/3
  Constant6/1 -> Shift Arithmetic12/1
  Bitwise Operator7/1 -> [RghtBsyBit3582]
  Shift Arithmetic15/1 -> Bitwise Operator7/1
  Shift Arithmetic14/1 -> Bitwise Operator7/2
  Shift Arithmetic13/1 -> Bitwise Operator7/3
  Constant8/1 -> Shift Arithmetic15/1
  Constant9/1 -> Shift Arithmetic14/1
  Constant10/1 -> Shift Arithmetic13/1
  [Is3582] -> Switch7/2
  Mux4/1 -> Switch7/1
  Mux5/1 -> Switch7/3
  [LftBsyBit3582] -> Mux4/1
  [RghtBsyBit3582] -> Mux4/2
  [LftBsyBit3582] -> Bitwise Operator8/1
  [RghtBsyBit3582] -> Bitwise Operator8/2
  Bitwise Operator8/1 -> [AllBsyBit3582]
  [AllBsyBit3582] -> Mux4/3
  [RghtBsyBit3582] -> Mux4/5
  [LftBsyBit3582] -> Mux4/4
  [RghtBsyBit3582] -> Mux4/6
  [LftBsyBit3582] -> Mux4/7
  Switch7/1 -> Demux/1
  [LftBsyBit] -> Mux5/1
  [RghtBsyBit] -> Mux5/2
  [LftBsyBit] -> Mux5/4
  [RghtBsyBit] -> Mux5/5
  Constant44/1 -> Mux5/3
  Constant45/1 -> Mux5/6
  Constant46/1 -> Mux5/7
  Demux/1 -> Mux3/3
  Demux/2 -> Mux3/4
  Demux/3 -> Mux3/5
  Demux/4 -> Mux3/6
  Demux/5 -> Mux3/7
  Demux/6 -> Mux3/8
  Demux/7 -> Mux3/9

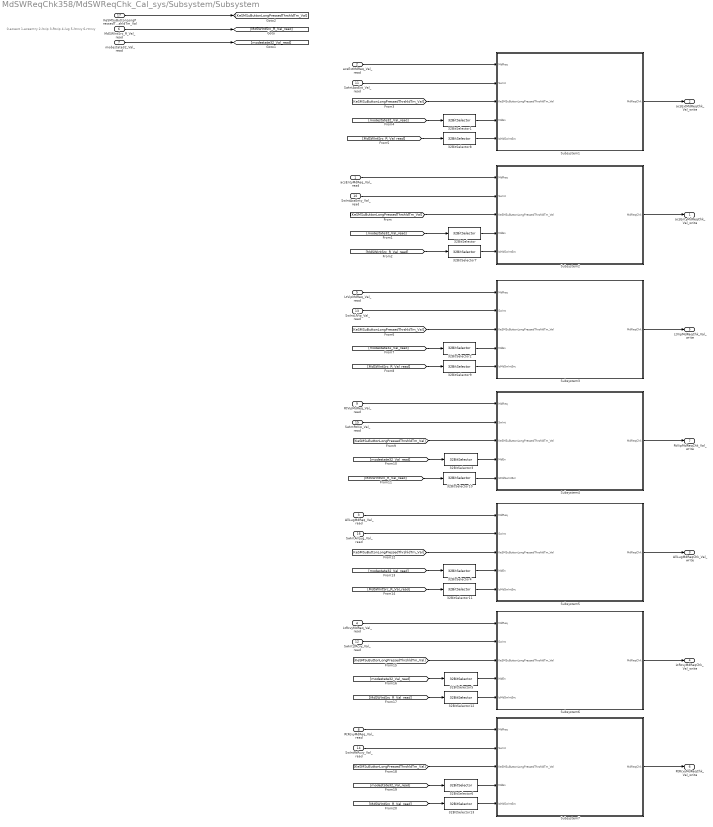
== system MdSWReqChk358/MdSWReqChk_Cal_sys/Subsystem/Subsystem ==
  note: 0-acsext 1-acsentry 2-ltvip 3-Rtvip 4-lug 5-ltrcvy 6-rtrcvy
  acsEntyMdReq_Val_read : Inport
  acsExtMdReq_Val_read : Inport  Port=2
  AllLugMdReq_Val_read : Inport  Port=3
  LtRcvyMdReq_Val_read : Inport  Port=4
  LtVipMdReq_Val_read : Inport  Port=5
  MdSWIntSrc_R_Val_read : Inport  Port=6
  modestate32_Val_read : Inport  Port=7
  RtRcvyMdReq_Val_read : Inport  Port=8
  RtVipMdReq_Val_read : Inport  Port=9
  SwIntAcsEnty_Val_read : Inport  Port=10
  SwIntAcsExt_Val_read : Inport  Port=11
  SwIntLfRcvy_Val_read : Inport  Port=12
  SwIntLfVip_Val_read : Inport  Port=13
  SwIntRtRcvy_Val_read : Inport  Port=14
  SwIntRtVip_Val_read : Inport  Port=15
  SwIntAllLug_Val_read : Inport  Port=16
  KeSMSuButtonLongPressedThrshldTm_Val : Inport  Port=17
  32BitSelector : RspLib/32BitSelector  BitNum=0
  32BitSelector1 : RspLib/32BitSelector  BitNum=3
  32BitSelector10 : RspLib/32BitSelector  BitNum=3
  32BitSelector11 : RspLib/32BitSelector  BitNum=4
  32BitSelector12 : RspLib/32BitSelector  BitNum=5
  32BitSelector13 : RspLib/32BitSelector  BitNum=6
  32BitSelector2 : RspLib/32BitSelector  BitNum=9
  32BitSelector3 : RspLib/32BitSelector  BitNum=11
  32BitSelector4 : RspLib/32BitSelector  BitNum=2
  32BitSelector5 : RspLib/32BitSelector  BitNum=10
  32BitSelector6 : RspLib/32BitSelector  BitNum=12
  32BitSelector7 : RspLib/32BitSelector  BitNum=1
  32BitSelector8 : RspLib/32BitSelector  BitNum=0
  32BitSelector9 : RspLib/32BitSelector  BitNum=2
  Subsystem1 : Subsystem
  Subsystem2 : Subsystem
  Subsystem3 : Subsystem
  Subsystem4 : Subsystem
  Subsystem5 : Subsystem
  Subsystem6 : Subsystem
  Subsystem7 : Subsystem
  acsEntyMdReqChk_Val_write : Outport
      settings: EnsureOutportIsVirtual=on
  acsExtMdReqChk_Val_write : Outport  Port=2
      settings: EnsureOutportIsVirtual=on
  AllLugMdReqChk_Val_write : Outport  Port=3
      settings: EnsureOutportIsVirtual=on
  LtRcvyMdReqChk_Val_write : Outport  Port=4
      settings: EnsureOutportIsVirtual=on
  LtVipMdReqChk_Val_write : Outport  Port=5
      settings: EnsureOutportIsVirtual=on
  RtRcvyMdReqChk_Val_write : Outport  Port=6
      settings: EnsureOutportIsVirtual=on
  RtVipMdReqChk_Val_write : Outport  Port=7
      settings: EnsureOutportIsVirtual=on
  wires:
  modestate32_Val_read/1 -> [modestate32_Val_read]
  SwIntAcsExt_Val_read/1 -> Subsystem1/2(SwInt)
  MdSWIntSrc_R_Val_read/1 -> [MdSWIntSrc_R_Val_read]
  SwIntAcsEnty_Val_read/1 -> Subsystem2/2(SwInt)
  KeSMSuButtonLongPressedThrshldTm_Val/1 -> [KeSMSuButtonLongPressedThrshldTm_Val]
  [KeSMSuButtonLongPressedThrshldTm_Val] -> Subsystem2/3(KeSMSuButtonLongPressedThrshldTm_Val)
  [modestate32_Val_read] -> 32BitSelector/1
  32BitSelector/1 -> Subsystem2/4(MdEn)
  [MdSWIntSrc_R_Val_read] -> 32BitSelector7/1
  32BitSelector7/1 -> Subsystem2/5(IsMdSwIntSrc)
  Subsystem2/1(MdReqChk) -> acsEntyMdReqChk_Val_write/1
  [KeSMSuButtonLongPressedThrshldTm_Val] -> Subsystem1/3(KeSMSuButtonLongPressedThrshldTm_Val)
  32BitSelector1/1 -> Subsystem1/4(MdEn)
  [modestate32_Val_read] -> 32BitSelector1/1
  32BitSelector8/1 -> Subsystem1/5(IsMdSwIntSrc)
  [MdSWIntSrc_R_Val_read] -> 32BitSelector8/1
  Subsystem1/1(MdReqChk) -> acsExtMdReqChk_Val_write/1
  acsExtMdReq_Val_read/1 -> Subsystem1/1(MdReq)
  acsEntyMdReq_Val_read/1 -> Subsystem2/1(MdReq)
  32BitSelector2/1 -> Subsystem3/4(MdEn)
  32BitSelector9/1 -> Subsystem3/5(IsMdSwIntSrc)
  [KeSMSuButtonLongPressedThrshldTm_Val] -> Subsystem3/3(KeSMSuButtonLongPressedThrshldTm_Val)
  [modestate32_Val_read] -> 32BitSelector2/1
  32BitSelector3/1 -> Subsystem4/4(MdEn)
  32BitSelector10/1 -> Subsystem4/5(IsMdSwIntSrc)
  [KeSMSuButtonLongPressedThrshldTm_Val] -> Subsystem4/3(KeSMSuButtonLongPressedThrshldTm_Val)
  [modestate32_Val_read] -> 32BitSelector3/1
  32BitSelector4/1 -> Subsystem5/4(MdEn)
  32BitSelector11/1 -> Subsystem5/5(IsMdSwIntSrc)
  [KeSMSuButtonLongPressedThrshldTm_Val] -> Subsystem5/3(KeSMSuButtonLongPressedThrshldTm_Val)
  [modestate32_Val_read] -> 32BitSelector4/1
  32BitSelector5/1 -> Subsystem6/4(MdEn)
  32BitSelector12/1 -> Subsystem6/5(IsMdSwIntSrc)
  [KeSMSuButtonLongPressedThrshldTm_Val] -> Subsystem6/3(KeSMSuButtonLongPressedThrshldTm_Val)
  [modestate32_Val_read] -> 32BitSelector5/1
  32BitSelector6/1 -> Subsystem7/4(MdEn)
  32BitSelector13/1 -> Subsystem7/5(IsMdSwIntSrc)
  [KeSMSuButtonLongPressedThrshldTm_Val] -> Subsystem7/3(KeSMSuButtonLongPressedThrshldTm_Val)
  [modestate32_Val_read] -> 32BitSelector6/1
  LtVipMdReq_Val_read/1 -> Subsystem3/1(MdReq)
  SwIntLfVip_Val_read/1 -> Subsystem3/2(SwInt)
  SwIntRtVip_Val_read/1 -> Subsystem4/2(SwInt)
  RtVipMdReq_Val_read/1 -> Subsystem4/1(MdReq)
  AllLugMdReq_Val_read/1 -> Subsystem5/1(MdReq)
  SwIntLfRcvy_Val_read/1 -> Subsystem6/2(SwInt)
  SwIntRtRcvy_Val_read/1 -> Subsystem7/2(SwInt)
  LtRcvyMdReq_Val_read/1 -> Subsystem6/1(MdReq)
  RtRcvyMdReq_Val_read/1 -> Subsystem7/1(MdReq)
  Subsystem3/1(MdReqChk) -> LtVipMdReqChk_Val_write/1
  Subsystem4/1(MdReqChk) -> RtVipMdReqChk_Val_write/1
  Subsystem5/1(MdReqChk) -> AllLugMdReqChk_Val_write/1
  Subsystem6/1(MdReqChk) -> LtRcvyMdReqChk_Val_write/1
  Subsystem7/1(MdReqChk) -> RtRcvyMdReqChk_Val_write/1
  SwIntAllLug_Val_read/1 -> Subsystem5/2(SwInt)
  [MdSWIntSrc_R_Val_read] -> 32BitSelector9/1
  [MdSWIntSrc_R_Val_read] -> 32BitSelector10/1
  [MdSWIntSrc_R_Val_read] -> 32BitSelector11/1
  [MdSWIntSrc_R_Val_read] -> 32BitSelector12/1
  [MdSWIntSrc_R_Val_read] -> 32BitSelector13/1

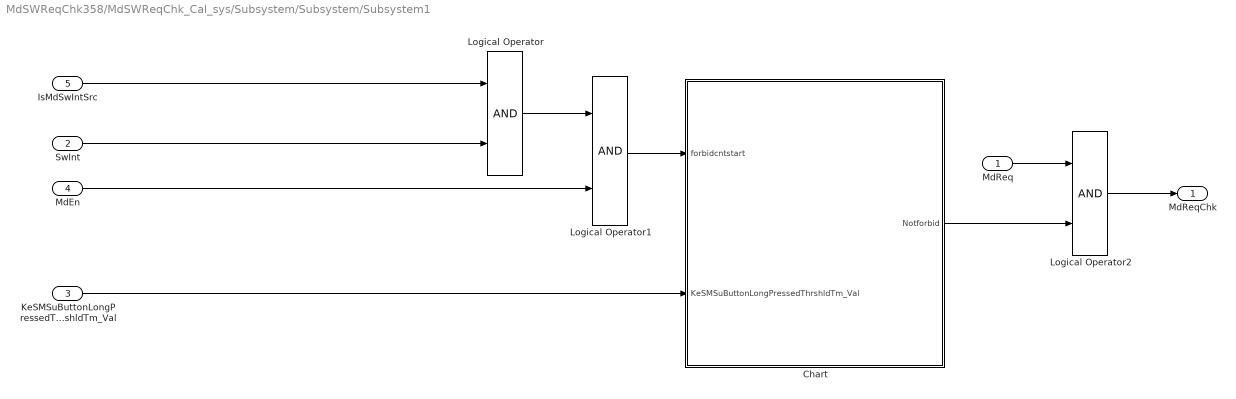
== system MdSWReqChk358/MdSWReqChk_Cal_sys/Subsystem/Subsystem/Subsystem1 ==
  MdReq : Inport
  SwInt : Inport  Port=2
  KeSMSuButtonLongPressedThrshldTm_Val : Inport  Port=3
  MdEn : Inport  Port=4
  IsMdSwIntSrc : Inport  Port=5
  Chart : Stateflow chart  TreatAsAtomicUnit=on
  Logical Operator : Logic  AllPortsSameDT=off  OutDataTypeStr=boolean
  Logical Operator1 : Logic  AllPortsSameDT=off  OutDataTypeStr=boolean
  Logical Operator2 : Logic  AllPortsSameDT=off  OutDataTypeStr=boolean
  MdReqChk : Outport
  wires:
  KeSMSuButtonLongPressedThrshldTm_Val/1 -> Chart/2(KeSMSuButtonLongPressedThrshldTm_Val)
  Logical Operator1/1 -> Chart/1(forbidcntstart)
  MdEn/1 -> Logical Operator1/2
  Logical Operator/1 -> Logical Operator1/1
  SwInt/1 -> Logical Operator/2
  IsMdSwIntSrc/1 -> Logical Operator/1
  Chart/1(Notforbid) -> Logical Operator2/2
  MdReq/1 -> Logical Operator2/1
  Logical Operator2/1 -> MdReqChk/1

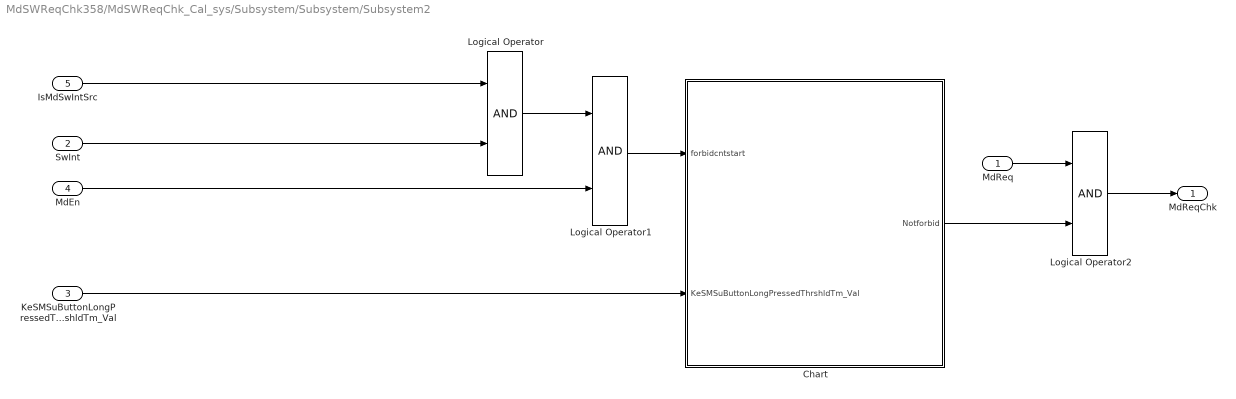
== system MdSWReqChk358/MdSWReqChk_Cal_sys/Subsystem/Subsystem/Subsystem2 ==
  MdReq : Inport
  SwInt : Inport  Port=2
  KeSMSuButtonLongPressedThrshldTm_Val : Inport  Port=3
  MdEn : Inport  Port=4
  IsMdSwIntSrc : Inport  Port=5
  Chart : Stateflow chart  TreatAsAtomicUnit=on
  Logical Operator : Logic  AllPortsSameDT=off  OutDataTypeStr=boolean
  Logical Operator1 : Logic  AllPortsSameDT=off  OutDataTypeStr=boolean
  Logical Operator2 : Logic  AllPortsSameDT=off  OutDataTypeStr=boolean
  MdReqChk : Outport
  wires:
  Logical Operator2/1 -> MdReqChk/1
  MdReq/1 -> Logical Operator2/1
  Chart/1(Notforbid) -> Logical Operator2/2
  IsMdSwIntSrc/1 -> Logical Operator/1
  SwInt/1 -> Logical Operator/2
  Logical Operator/1 -> Logical Operator1/1
  MdEn/1 -> Logical Operator1/2
  Logical Operator1/1 -> Chart/1(forbidcntstart)
  KeSMSuButtonLongPressedThrshldTm_Val/1 -> Chart/2(KeSMSuButtonLongPressedThrshldTm_Val)

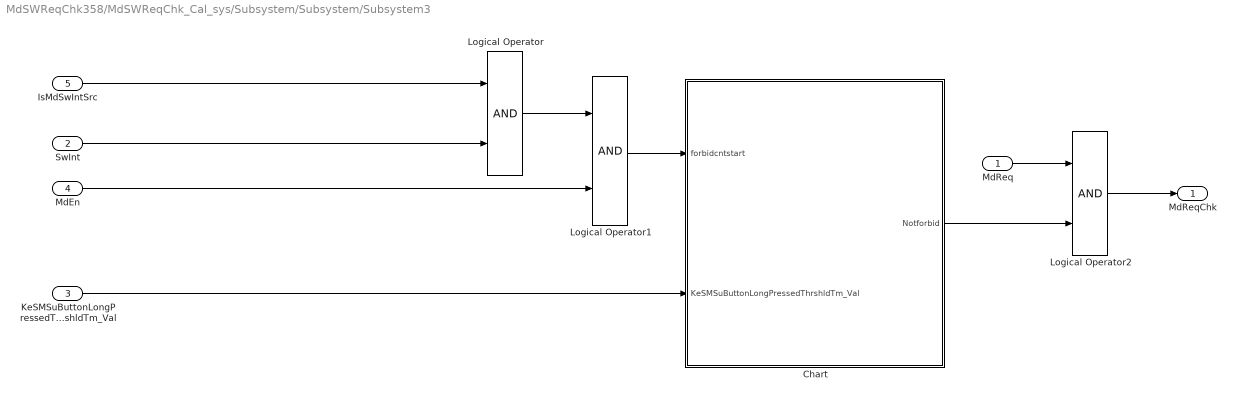
== system MdSWReqChk358/MdSWReqChk_Cal_sys/Subsystem/Subsystem/Subsystem3 ==
  MdReq : Inport
  SwInt : Inport  Port=2
  KeSMSuButtonLongPressedThrshldTm_Val : Inport  Port=3
  MdEn : Inport  Port=4
  IsMdSwIntSrc : Inport  Port=5
  Chart : Stateflow chart  TreatAsAtomicUnit=on
  Logical Operator : Logic  AllPortsSameDT=off  OutDataTypeStr=boolean
  Logical Operator1 : Logic  AllPortsSameDT=off  OutDataTypeStr=boolean
  Logical Operator2 : Logic  AllPortsSameDT=off  OutDataTypeStr=boolean
  MdReqChk : Outport
  wires:
  Logical Operator2/1 -> MdReqChk/1
  MdReq/1 -> Logical Operator2/1
  Chart/1(Notforbid) -> Logical Operator2/2
  IsMdSwIntSrc/1 -> Logical Operator/1
  SwInt/1 -> Logical Operator/2
  Logical Operator/1 -> Logical Operator1/1
  MdEn/1 -> Logical Operator1/2
  Logical Operator1/1 -> Chart/1(forbidcntstart)
  KeSMSuButtonLongPressedThrshldTm_Val/1 -> Chart/2(KeSMSuButtonLongPressedThrshldTm_Val)

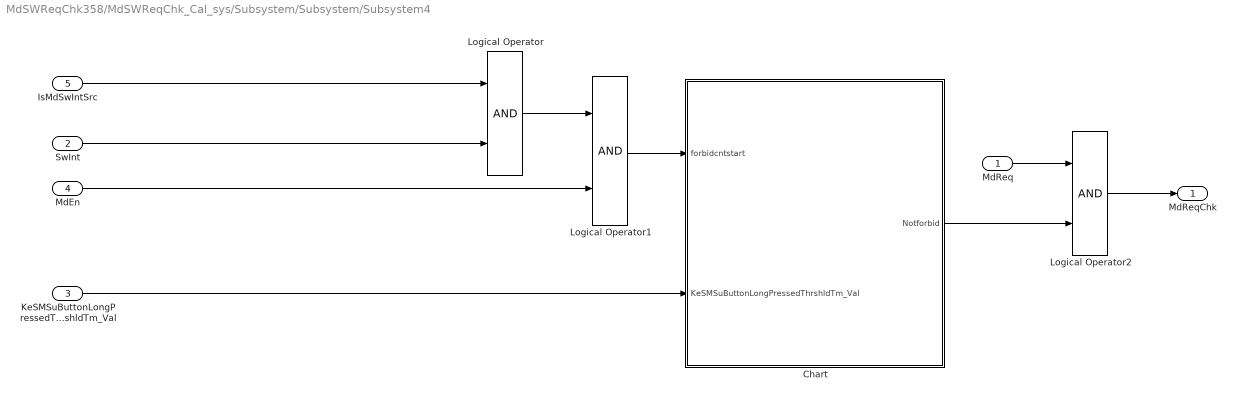
== system MdSWReqChk358/MdSWReqChk_Cal_sys/Subsystem/Subsystem/Subsystem4 ==
  MdReq : Inport
  SwInt : Inport  Port=2
  KeSMSuButtonLongPressedThrshldTm_Val : Inport  Port=3
  MdEn : Inport  Port=4
  IsMdSwIntSrc : Inport  Port=5
  Chart : Stateflow chart  TreatAsAtomicUnit=on
  Logical Operator : Logic  AllPortsSameDT=off  OutDataTypeStr=boolean
  Logical Operator1 : Logic  AllPortsSameDT=off  OutDataTypeStr=boolean
  Logical Operator2 : Logic  AllPortsSameDT=off  OutDataTypeStr=boolean
  MdReqChk : Outport
  wires:
  KeSMSuButtonLongPressedThrshldTm_Val/1 -> Chart/2(KeSMSuButtonLongPressedThrshldTm_Val)
  Logical Operator1/1 -> Chart/1(forbidcntstart)
  MdEn/1 -> Logical Operator1/2
  Logical Operator/1 -> Logical Operator1/1
  SwInt/1 -> Logical Operator/2
  IsMdSwIntSrc/1 -> Logical Operator/1
  Chart/1(Notforbid) -> Logical Operator2/2
  MdReq/1 -> Logical Operator2/1
  Logical Operator2/1 -> MdReqChk/1

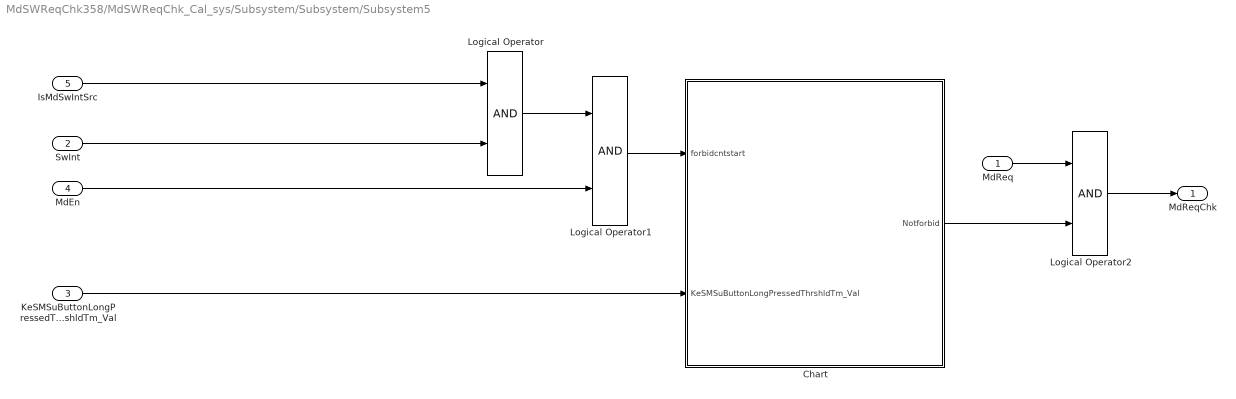
== system MdSWReqChk358/MdSWReqChk_Cal_sys/Subsystem/Subsystem/Subsystem5 ==
  MdReq : Inport
  SwInt : Inport  Port=2
  KeSMSuButtonLongPressedThrshldTm_Val : Inport  Port=3
  MdEn : Inport  Port=4
  IsMdSwIntSrc : Inport  Port=5
  Chart : Stateflow chart  TreatAsAtomicUnit=on
  Logical Operator : Logic  AllPortsSameDT=off  OutDataTypeStr=boolean
  Logical Operator1 : Logic  AllPortsSameDT=off  OutDataTypeStr=boolean
  Logical Operator2 : Logic  AllPortsSameDT=off  OutDataTypeStr=boolean
  MdReqChk : Outport
  wires:
  Logical Operator2/1 -> MdReqChk/1
  MdReq/1 -> Logical Operator2/1
  Chart/1(Notforbid) -> Logical Operator2/2
  IsMdSwIntSrc/1 -> Logical Operator/1
  SwInt/1 -> Logical Operator/2
  Logical Operator/1 -> Logical Operator1/1
  MdEn/1 -> Logical Operator1/2
  Logical Operator1/1 -> Chart/1(forbidcntstart)
  KeSMSuButtonLongPressedThrshldTm_Val/1 -> Chart/2(KeSMSuButtonLongPressedThrshldTm_Val)

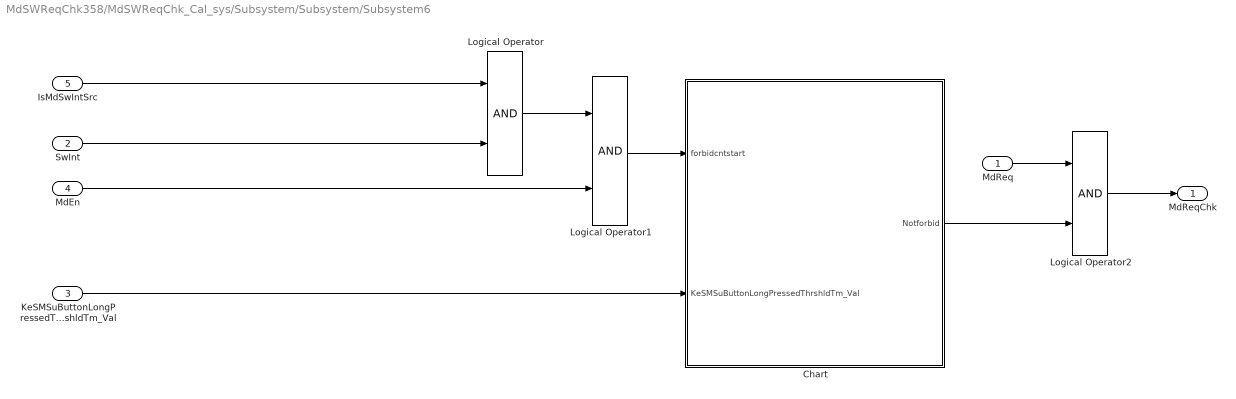
== system MdSWReqChk358/MdSWReqChk_Cal_sys/Subsystem/Subsystem/Subsystem6 ==
  MdReq : Inport
  SwInt : Inport  Port=2
  KeSMSuButtonLongPressedThrshldTm_Val : Inport  Port=3
  MdEn : Inport  Port=4
  IsMdSwIntSrc : Inport  Port=5
  Chart : Stateflow chart  TreatAsAtomicUnit=on
  Logical Operator : Logic  AllPortsSameDT=off  OutDataTypeStr=boolean
  Logical Operator1 : Logic  AllPortsSameDT=off  OutDataTypeStr=boolean
  Logical Operator2 : Logic  AllPortsSameDT=off  OutDataTypeStr=boolean
  MdReqChk : Outport
  wires:
  KeSMSuButtonLongPressedThrshldTm_Val/1 -> Chart/2(KeSMSuButtonLongPressedThrshldTm_Val)
  Logical Operator1/1 -> Chart/1(forbidcntstart)
  MdEn/1 -> Logical Operator1/2
  Logical Operator/1 -> Logical Operator1/1
  SwInt/1 -> Logical Operator/2
  IsMdSwIntSrc/1 -> Logical Operator/1
  Chart/1(Notforbid) -> Logical Operator2/2
  MdReq/1 -> Logical Operator2/1
  Logical Operator2/1 -> MdReqChk/1

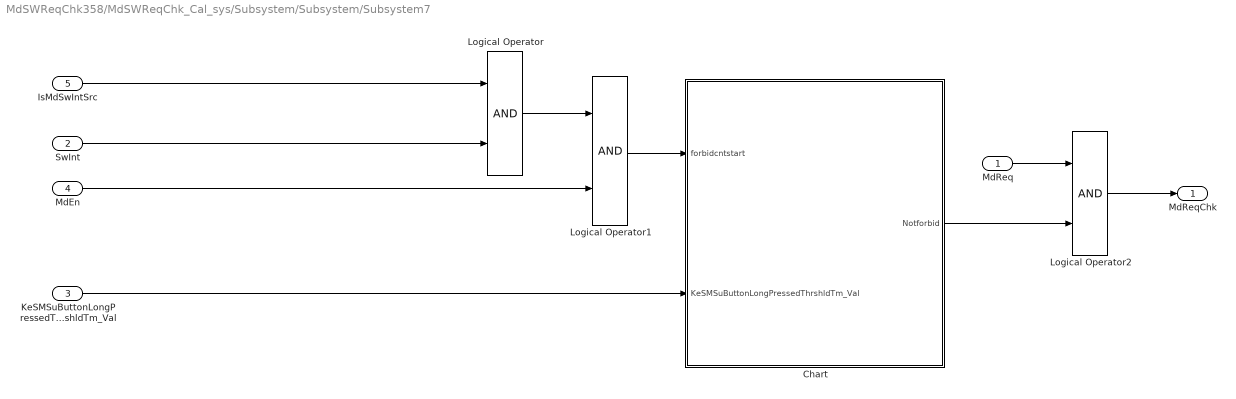
== system MdSWReqChk358/MdSWReqChk_Cal_sys/Subsystem/Subsystem/Subsystem7 ==
  MdReq : Inport
  SwInt : Inport  Port=2
  KeSMSuButtonLongPressedThrshldTm_Val : Inport  Port=3
  MdEn : Inport  Port=4
  IsMdSwIntSrc : Inport  Port=5
  Chart : Stateflow chart  TreatAsAtomicUnit=on
  Logical Operator : Logic  AllPortsSameDT=off  OutDataTypeStr=boolean
  Logical Operator1 : Logic  AllPortsSameDT=off  OutDataTypeStr=boolean
  Logical Operator2 : Logic  AllPortsSameDT=off  OutDataTypeStr=boolean
  MdReqChk : Outport
  wires:
  Logical Operator2/1 -> MdReqChk/1
  MdReq/1 -> Logical Operator2/1
  Chart/1(Notforbid) -> Logical Operator2/2
  IsMdSwIntSrc/1 -> Logical Operator/1
  SwInt/1 -> Logical Operator/2
  Logical Operator/1 -> Logical Operator1/1
  MdEn/1 -> Logical Operator1/2
  Logical Operator1/1 -> Chart/1(forbidcntstart)
  KeSMSuButtonLongPressedThrshldTm_Val/1 -> Chart/2(KeSMSuButtonLongPressedThrshldTm_Val)

== stateflow chart MdSWReqChk358/MdSWReqChk_Cal_sys/Subsystem/Subsystem/Subsystem1/Chart ==
  state fobidStop
    en:Notforbid = true;
  state fobidCntStart
    en:forbidcnt=1;
    du:forbidcnt=forbidcnt+1;
  state fobid
    en:Notforbid=false;
    en:forbidcnt=1;
    du:forbidcnt=forbidcnt+1;
  (default) -> fobidStop
  fobidStop -> fobidCntStart : [forbidcntstart]
  fobidCntStart -> fobid : [forbidcnt>=(KeSMSuButtonLongPressedThrshldTm_Val-5)]
  fobid -> fobidStop : [forbidcnt >10]
  data: forbidcntstart input boolean; forbidcnt local uint8; KeSMSuButtonLongPressedThrshldTm_Val input; Notforbid output boolean

== stateflow chart MdSWReqChk358/MdSWReqChk_Cal_sys/Subsystem/Subsystem/Subsystem2/Chart ==
  state fobidStop
    en:Notforbid = true;
  state fobidCntStart
    en:forbidcnt=1;
    du:forbidcnt=forbidcnt+1;
  state fobid
    en:Notforbid=false;
    en:forbidcnt=1;
    du:forbidcnt=forbidcnt+1;
  (default) -> fobidStop
  fobidStop -> fobidCntStart : [forbidcntstart]
  fobidCntStart -> fobid : [forbidcnt>=(KeSMSuButtonLongPressedThrshldTm_Val-5)]
  fobid -> fobidStop : [forbidcnt >10]
  data: forbidcntstart input boolean; forbidcnt local uint8; KeSMSuButtonLongPressedThrshldTm_Val input; Notforbid output boolean

== stateflow chart MdSWReqChk358/MdSWReqChk_Cal_sys/Subsystem/Subsystem/Subsystem3/Chart ==
  state fobidStop
    en:Notforbid = true;
  state fobidCntStart
    en:forbidcnt=1;
    du:forbidcnt=forbidcnt+1;
  state fobid
    en:Notforbid=false;
    en:forbidcnt=1;
    du:forbidcnt=forbidcnt+1;
  (default) -> fobidStop
  fobidStop -> fobidCntStart : [forbidcntstart]
  fobidCntStart -> fobid : [forbidcnt>=(KeSMSuButtonLongPressedThrshldTm_Val-5)]
  fobid -> fobidStop : [forbidcnt >10]
  data: forbidcntstart input boolean; forbidcnt local uint8; KeSMSuButtonLongPressedThrshldTm_Val input; Notforbid output boolean

== stateflow chart MdSWReqChk358/MdSWReqChk_Cal_sys/Subsystem/Subsystem/Subsystem4/Chart ==
  state fobidStop
    en:Notforbid = true;
  state fobidCntStart
    en:forbidcnt=1;
    du:forbidcnt=forbidcnt+1;
  state fobid
    en:Notforbid=false;
    en:forbidcnt=1;
    du:forbidcnt=forbidcnt+1;
  (default) -> fobidStop
  fobidStop -> fobidCntStart : [forbidcntstart]
  fobidCntStart -> fobid : [forbidcnt>=(KeSMSuButtonLongPressedThrshldTm_Val-5)]
  fobid -> fobidStop : [forbidcnt >10]
  data: forbidcntstart input boolean; forbidcnt local uint8; KeSMSuButtonLongPressedThrshldTm_Val input; Notforbid output boolean

== stateflow chart MdSWReqChk358/MdSWReqChk_Cal_sys/Subsystem/Subsystem/Subsystem5/Chart ==
  state fobidStop
    en:Notforbid = true;
  state fobidCntStart
    en:forbidcnt=1;
    du:forbidcnt=forbidcnt+1;
  state fobid
    en:Notforbid=false;
    en:forbidcnt=1;
    du:forbidcnt=forbidcnt+1;
  (default) -> fobidStop
  fobidStop -> fobidCntStart : [forbidcntstart]
  fobidCntStart -> fobid : [forbidcnt>=(KeSMSuButtonLongPressedThrshldTm_Val-5)]
  fobid -> fobidStop : [forbidcnt >10]
  data: forbidcntstart input boolean; forbidcnt local uint8; KeSMSuButtonLongPressedThrshldTm_Val input; Notforbid output boolean

== stateflow chart MdSWReqChk358/MdSWReqChk_Cal_sys/Subsystem/Subsystem/Subsystem6/Chart ==
  state fobidStop
    en:Notforbid = true;
  state fobidCntStart
    en:forbidcnt=1;
    du:forbidcnt=forbidcnt+1;
  state fobid
    en:Notforbid=false;
    en:forbidcnt=1;
    du:forbidcnt=forbidcnt+1;
  (default) -> fobidStop
  fobidStop -> fobidCntStart : [forbidcntstart]
  fobidCntStart -> fobid : [forbidcnt>=(KeSMSuButtonLongPressedThrshldTm_Val-5)]
  fobid -> fobidStop : [forbidcnt >10]
  data: forbidcntstart input boolean; forbidcnt local uint8; KeSMSuButtonLongPressedThrshldTm_Val input; Notforbid output boolean

== stateflow chart MdSWReqChk358/MdSWReqChk_Cal_sys/Subsystem/Subsystem/Subsystem7/Chart ==
  state fobidStop
    en:Notforbid = true;
  state fobidCntStart
    en:forbidcnt=1;
    du:forbidcnt=forbidcnt+1;
  state fobid
    en:Notforbid=false;
    en:forbidcnt=1;
    du:forbidcnt=forbidcnt+1;
  (default) -> fobidStop
  fobidStop -> fobidCntStart : [forbidcntstart]
  fobidCntStart -> fobid : [forbidcnt>=(KeSMSuButtonLongPressedThrshldTm_Val-5)]
  fobid -> fobidStop : [forbidcnt >10]
  data: forbidcntstart input boolean; forbidcnt local uint8; KeSMSuButtonLongPressedThrshldTm_Val input; Notforbid output boolean
